simulink model "kb1ram"  (R2020a)
settings: Solver=VariableStepAuto  StartTime=0.0  StopTime=10.0  RelTol=1e-3
libraries: simulink_extras x10
settings Model: Creator=kishan  LastModifiedBy=kishan

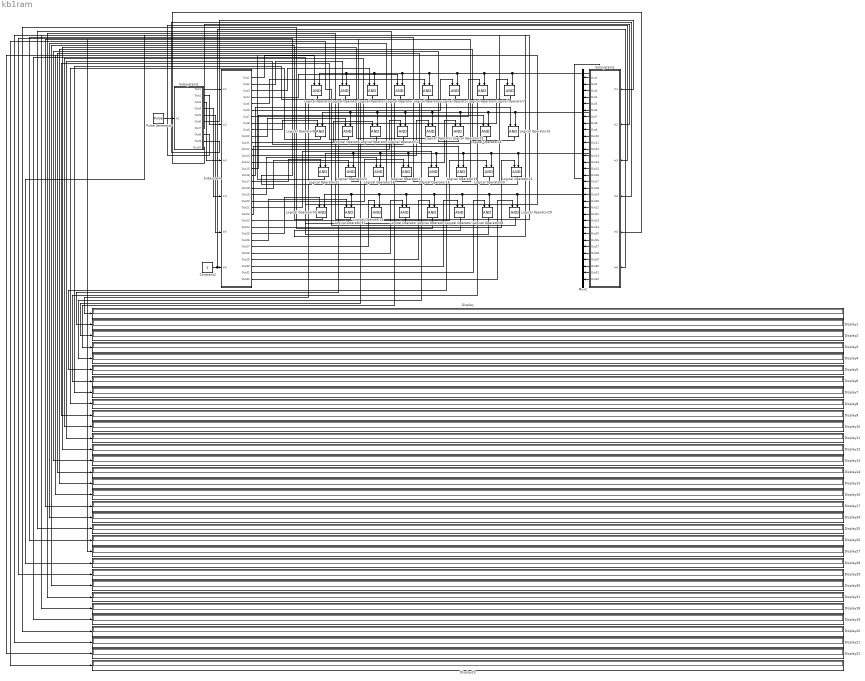
== system kb1ram ==
  Constant2 : Constant
  Display{,1..31} (32 alike) : Display
  Logical Operator{,1..31} (32 alike) : Logic  AllPortsSameDT=off  OutDataTypeStr=boolean
  Mux2 : Mux  Inputs=32
  Pulse Generator : DiscretePulseGenerator  PulseType=Time based  Period=0.005  PulseWidth=5
  Subsystem : Subsystem
  Subsystem1 : Subsystem
  Subsystem2 : Subsystem
  wires:
  Subsystem1/1(Out1) -> Mux2/1
  Subsystem1/2(Out2) -> Mux2/2
  Subsystem1/3(Out3) -> Mux2/3
  Subsystem1/4(Out4) -> Mux2/4
  Subsystem1/5(Out5) -> Mux2/5
  Subsystem1/6(Out6) -> Mux2/6
  Subsystem1/7(Out7) -> Mux2/7
  Subsystem1/8(Out8) -> Mux2/8
  Subsystem1/9(Out9) -> Mux2/9
  Subsystem1/10(Out10) -> Mux2/10
  Subsystem1/11(Out11) -> Mux2/11
  Subsystem1/12(Out12) -> Mux2/12
  Subsystem1/13(Out13) -> Mux2/13
  Subsystem1/14(Out14) -> Mux2/14
  Subsystem1/15(Out15) -> Mux2/15
  Subsystem1/16(Out16) -> Mux2/16
  Subsystem1/17(Out17) -> Mux2/17
  Subsystem1/18(Out18) -> Mux2/18
  Subsystem1/19(Out19) -> Mux2/19
  Subsystem1/20(Out20) -> Mux2/20
  Subsystem1/21(Out21) -> Mux2/21
  Subsystem1/22(Out22) -> Mux2/22
  Subsystem1/23(Out23) -> Mux2/23
  Subsystem1/24(Out24) -> Mux2/24
  Subsystem1/25(Out25) -> Mux2/25
  Subsystem1/26(Out26) -> Mux2/26
  Subsystem1/27(Out27) -> Mux2/27
  Subsystem1/28(Out28) -> Mux2/28
  Subsystem1/29(Out29) -> Mux2/29
  Subsystem1/30(Out30) -> Mux2/30
  Subsystem1/31(Out31) -> Mux2/31
  Subsystem1/32(Out32) -> Mux2/32
  Subsystem2/1(Out1) -> Subsystem/1(In1)
  Subsystem2/2(Out2) -> Subsystem/2(In2)
  Subsystem2/5(Out5) -> Subsystem/5(In5)
  Subsystem2/4(Out4) -> Subsystem/4(In4)
  Subsystem2/3(Out3) -> Subsystem/3(In3)
  Subsystem2/6(Out6) -> Subsystem1/1(In1)
  Subsystem2/7(Out7) -> Subsystem1/2(In2)
  Subsystem2/8(Out8) -> Subsystem1/3(In3)
  Constant2/1 -> Subsystem1/6(In6), Subsystem/6(In6)
  Subsystem2/10(Out10) -> Subsystem1/5(In5)
  Subsystem2/9(Out9) -> Subsystem1/4(In4)
  Subsystem/1(Out1) -> Logical Operator/1
  Subsystem/2(Out2) -> Logical Operator1/1
  Subsystem/3(Out3) -> Logical Operator2/1
  Subsystem/4(Out4) -> Logical Operator3/1
  Mux2/1 -> Logical Operator31/2, Logical Operator30/2, Logical Operator24/2, Logical Operator25/2, Logical Operator26/2, Logical Operator27/2, Logical Operator28/2, Logical Operator29/2, Logical Operator21/2, Logical Operator23/2, Logical Operator22/2, Logical Operator16/2, Logical Operator17/2, Logical Operator18/2, Logical Operator19/2, Logical Operator20/2, Logical Operator9/2, Logical Operator8/2, Logical Operator10/2, Logical Operator11/2, Logical Operator12/2, Logical Operator13/2, Logical Operator14/2, Logical Operator15/2, Logical Operator1/2, Logical Operator/2, Logical Operator2/2, Logical Operator3/2, Logical Operator4/2, Logical Operator5/2, Logical Operator6/2, Logical Operator7/2
  Subsystem/5(Out5) -> Logical Operator4/1
  Subsystem/6(Out6) -> Logical Operator5/1
  Subsystem/7(Out7) -> Logical Operator6/1
  Subsystem/8(Out8) -> Logical Operator7/1
  Subsystem/9(Out9) -> Logical Operator8/1
  Subsystem/10(Out10) -> Logical Operator9/1
  Subsystem/11(Out11) -> Logical Operator10/1
  Subsystem/12(Out12) -> Logical Operator11/1
  Subsystem/13(Out13) -> Logical Operator12/1
  Subsystem/14(Out14) -> Logical Operator13/1
  Subsystem/15(Out15) -> Logical Operator14/1
  Subsystem/16(Out16) -> Logical Operator15/1
  Subsystem/17(Out17) -> Logical Operator22/1
  Subsystem/18(Out18) -> Logical Operator23/1
  Subsystem/19(Out19) -> Logical Operator16/1
  Subsystem/20(Out20) -> Logical Operator17/1
  Subsystem/21(Out21) -> Logical Operator18/1
  Subsystem/22(Out22) -> Logical Operator19/1
  Subsystem/23(Out23) -> Logical Operator20/1
  Subsystem/24(Out24) -> Logical Operator21/1
  Subsystem/25(Out25) -> Logical Operator30/1
  Subsystem/26(Out26) -> Logical Operator31/1
  Subsystem/27(Out27) -> Logical Operator24/1
  Subsystem/28(Out28) -> Logical Operator25/1
  Subsystem/29(Out29) -> Logical Operator26/1
  Subsystem/30(Out30) -> Logical Operator27/1
  Subsystem/31(Out31) -> Logical Operator28/1
  Subsystem/32(Out32) -> Logical Operator29/1
  Logical Operator/1 -> Display/1
  Logical Operator1/1 -> Display1/1
  Logical Operator2/1 -> Display2/1
  Logical Operator3/1 -> Display3/1
  Logical Operator4/1 -> Display4/1
  Logical Operator5/1 -> Display5/1
  Logical Operator6/1 -> Display6/1
  Logical Operator7/1 -> Display7/1
  Logical Operator8/1 -> Display8/1
  Logical Operator9/1 -> Display9/1
  Logical Operator10/1 -> Display10/1
  Logical Operator11/1 -> Display11/1
  Logical Operator12/1 -> Display12/1
  Logical Operator13/1 -> Display13/1
  Logical Operator14/1 -> Display14/1
  Logical Operator15/1 -> Display15/1
  Logical Operator17/1 -> Display25/1
  Logical Operator30/1 -> Display30/1
  Logical Operator22/1 -> Display16/1
  Logical Operator26/1 -> Display20/1
  Logical Operator27/1 -> Display21/1
  Logical Operator18/1 -> Display26/1
  Logical Operator29/1 -> Display23/1
  Logical Operator31/1 -> Display31/1
  Logical Operator25/1 -> Display19/1
  Logical Operator19/1 -> Display27/1
  Logical Operator28/1 -> Display22/1
  Logical Operator21/1 -> Display29/1
  Logical Operator24/1 -> Display18/1
  Logical Operator16/1 -> Display24/1
  Logical Operator20/1 -> Display28/1
  Logical Operator23/1 -> Display17/1
  Pulse Generator/1 -> Subsystem2/1(In1)

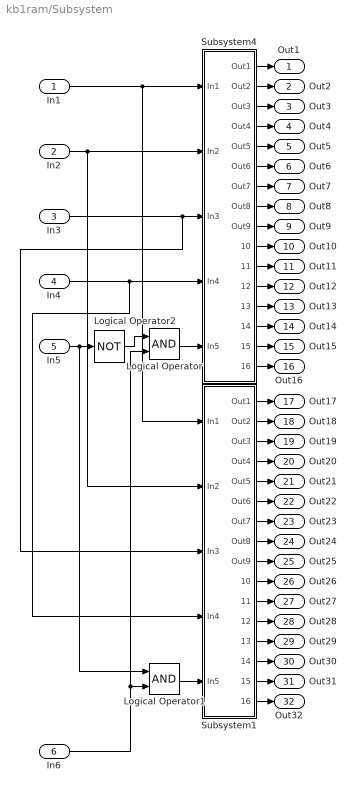
== system kb1ram/Subsystem ==
  In1 : Inport
  In2 : Inport  Port=2
  In3 : Inport  Port=3
  In4 : Inport  Port=4
  In5 : Inport  Port=5
  In6 : Inport  Port=6
  Logical Operator : Logic  AllPortsSameDT=off  OutDataTypeStr=boolean
  Logical Operator1 : Logic  AllPortsSameDT=off  OutDataTypeStr=boolean
  Logical Operator2 : Logic  Operator=NOT  AllPortsSameDT=off  OutDataTypeStr=boolean
  Subsystem1 : Subsystem
  Subsystem4 : Subsystem
  Out1 : Outport
  Out2 : Outport  Port=2
  Out3 : Outport  Port=3
  Out4 : Outport  Port=4
  Out5 : Outport  Port=5
  Out6 : Outport  Port=6
  Out7 : Outport  Port=7
  Out8 : Outport  Port=8
  Out9 : Outport  Port=9
  Out10 : Outport  Port=10
  Out11 : Outport  Port=11
  Out12 : Outport  Port=12
  Out13 : Outport  Port=13
  Out14 : Outport  Port=14
  Out15 : Outport  Port=15
  Out16 : Outport  Port=16
  Out17 : Outport  Port=17
  Out18 : Outport  Port=18
  Out19 : Outport  Port=19
  Out20 : Outport  Port=20
  Out21 : Outport  Port=21
  Out22 : Outport  Port=22
  Out23 : Outport  Port=23
  Out24 : Outport  Port=24
  Out25 : Outport  Port=25
  Out26 : Outport  Port=26
  Out27 : Outport  Port=27
  Out28 : Outport  Port=28
  Out29 : Outport  Port=29
  Out30 : Outport  Port=30
  Out31 : Outport  Port=31
  Out32 : Outport  Port=32
  wires:
  Subsystem1/3(Out3) -> Out19/1
  Subsystem4/2(Out2) -> Out2/1
  Logical Operator2/1 -> Logical Operator/1
  Subsystem4/4(Out4) -> Out4/1
  Subsystem4/11(Out11) -> Out11/1
  Subsystem1/13(Out13) -> Out29/1
  Subsystem4/9(Out9) -> Out9/1
  Subsystem4/13(Out13) -> Out13/1
  Subsystem4/7(Out7) -> Out7/1
  Subsystem1/12(Out12) -> Out28/1
  Subsystem4/6(Out6) -> Out6/1
  Subsystem1/14(Out14) -> Out30/1
  Logical Operator1/1 -> Subsystem1/5(In5)
  Subsystem4/5(Out5) -> Out5/1
  Subsystem1/9(Out9) -> Out25/1
  Subsystem4/10(Out10) -> Out10/1
  Subsystem4/8(Out8) -> Out8/1
  In6/1 -> Logical Operator/2, Logical Operator1/2
  Subsystem1/4(Out4) -> Out20/1
  Subsystem1/15(Out15) -> Out31/1
  In1/1 -> Subsystem4/1(In1), Subsystem1/1(In1)
  Subsystem1/6(Out6) -> Out22/1
  Subsystem1/10(Out10) -> Out26/1
  Subsystem1/11(Out11) -> Out27/1
  Subsystem1/2(Out2) -> Out18/1
  Subsystem1/7(Out7) -> Out23/1
  Subsystem4/1(Out1) -> Out1/1
  Subsystem1/16(Out16) -> Out32/1
  Subsystem1/1(Out1) -> Out17/1
  Subsystem4/12(Out12) -> Out12/1
  In4/1 -> Subsystem1/4(In4), Subsystem4/4(In4)
  Subsystem1/8(Out8) -> Out24/1
  In2/1 -> Subsystem4/2(In2), Subsystem1/2(In2)
  In5/1 -> Logical Operator1/1, Logical Operator2/1
  Subsystem4/3(Out3) -> Out3/1
  Subsystem4/15(Out15) -> Out15/1
  Subsystem4/16(Out16) -> Out16/1
  Subsystem1/5(Out5) -> Out21/1
  Subsystem4/14(Out14) -> Out14/1
  In3/1 -> Subsystem1/3(In3), Subsystem4/3(In3)
  Logical Operator/1 -> Subsystem4/5(In5)

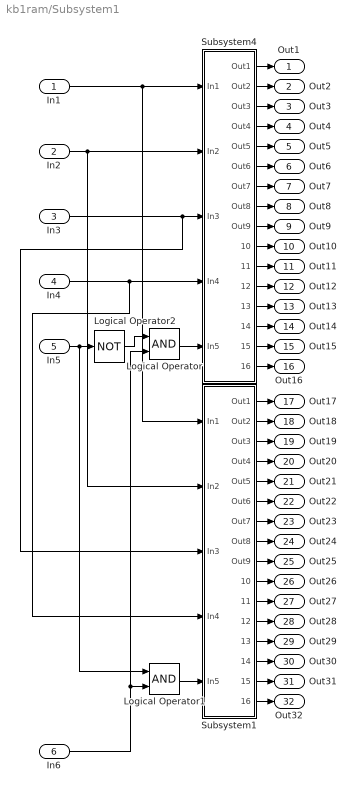
== system kb1ram/Subsystem1 ==
  In1 : Inport
  In2 : Inport  Port=2
  In3 : Inport  Port=3
  In4 : Inport  Port=4
  In5 : Inport  Port=5
  In6 : Inport  Port=6
  Logical Operator : Logic  AllPortsSameDT=off  OutDataTypeStr=boolean
  Logical Operator1 : Logic  AllPortsSameDT=off  OutDataTypeStr=boolean
  Logical Operator2 : Logic  Operator=NOT  AllPortsSameDT=off  OutDataTypeStr=boolean
  Subsystem1 : Subsystem
  Subsystem4 : Subsystem
  Out1 : Outport
  Out2 : Outport  Port=2
  Out3 : Outport  Port=3
  Out4 : Outport  Port=4
  Out5 : Outport  Port=5
  Out6 : Outport  Port=6
  Out7 : Outport  Port=7
  Out8 : Outport  Port=8
  Out9 : Outport  Port=9
  Out10 : Outport  Port=10
  Out11 : Outport  Port=11
  Out12 : Outport  Port=12
  Out13 : Outport  Port=13
  Out14 : Outport  Port=14
  Out15 : Outport  Port=15
  Out16 : Outport  Port=16
  Out17 : Outport  Port=17
  Out18 : Outport  Port=18
  Out19 : Outport  Port=19
  Out20 : Outport  Port=20
  Out21 : Outport  Port=21
  Out22 : Outport  Port=22
  Out23 : Outport  Port=23
  Out24 : Outport  Port=24
  Out25 : Outport  Port=25
  Out26 : Outport  Port=26
  Out27 : Outport  Port=27
  Out28 : Outport  Port=28
  Out29 : Outport  Port=29
  Out30 : Outport  Port=30
  Out31 : Outport  Port=31
  Out32 : Outport  Port=32
  wires:
  Subsystem1/3(Out3) -> Out19/1
  Subsystem4/2(Out2) -> Out2/1
  Logical Operator2/1 -> Logical Operator/1
  Subsystem4/4(Out4) -> Out4/1
  Subsystem4/11(Out11) -> Out11/1
  Subsystem1/13(Out13) -> Out29/1
  Subsystem4/9(Out9) -> Out9/1
  Subsystem4/13(Out13) -> Out13/1
  Subsystem4/7(Out7) -> Out7/1
  Subsystem1/12(Out12) -> Out28/1
  Subsystem4/6(Out6) -> Out6/1
  Subsystem1/14(Out14) -> Out30/1
  Logical Operator1/1 -> Subsystem1/5(In5)
  Subsystem4/5(Out5) -> Out5/1
  Subsystem1/9(Out9) -> Out25/1
  Subsystem4/10(Out10) -> Out10/1
  Subsystem4/8(Out8) -> Out8/1
  In6/1 -> Logical Operator/2, Logical Operator1/2
  Subsystem1/4(Out4) -> Out20/1
  Subsystem1/15(Out15) -> Out31/1
  In1/1 -> Subsystem4/1(In1), Subsystem1/1(In1)
  Subsystem1/6(Out6) -> Out22/1
  Subsystem1/10(Out10) -> Out26/1
  Subsystem1/11(Out11) -> Out27/1
  Subsystem1/2(Out2) -> Out18/1
  Subsystem1/7(Out7) -> Out23/1
  Subsystem4/1(Out1) -> Out1/1
  Subsystem1/16(Out16) -> Out32/1
  Subsystem1/1(Out1) -> Out17/1
  Subsystem4/12(Out12) -> Out12/1
  In4/1 -> Subsystem1/4(In4), Subsystem4/4(In4)
  Subsystem1/8(Out8) -> Out24/1
  In2/1 -> Subsystem4/2(In2), Subsystem1/2(In2)
  In5/1 -> Logical Operator1/1, Logical Operator2/1
  Subsystem4/3(Out3) -> Out3/1
  Subsystem4/15(Out15) -> Out15/1
  Subsystem4/16(Out16) -> Out16/1
  Subsystem1/5(Out5) -> Out21/1
  Subsystem4/14(Out14) -> Out14/1
  In3/1 -> Subsystem1/3(In3), Subsystem4/3(In3)
  Logical Operator/1 -> Subsystem4/5(In5)

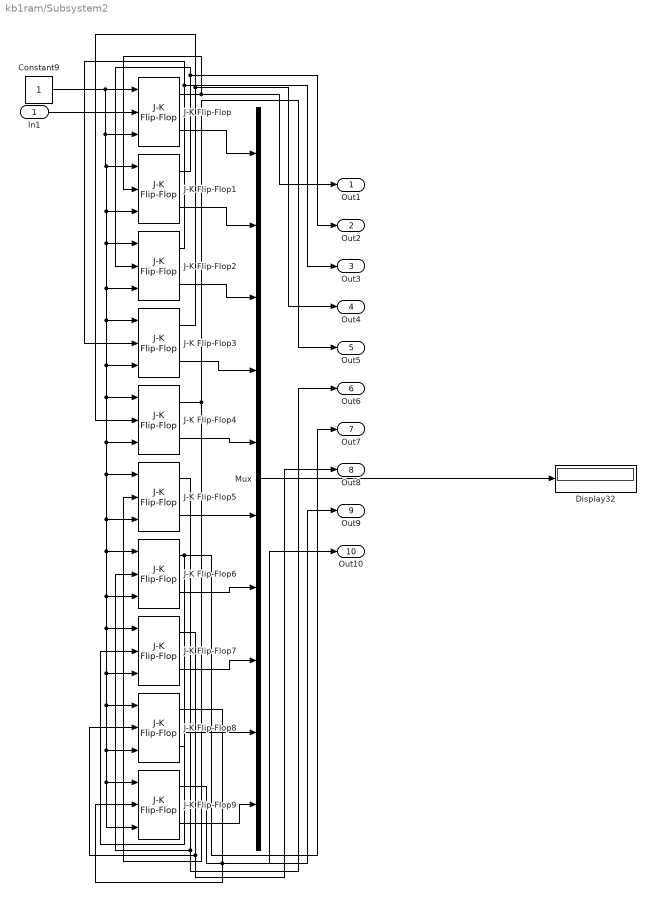
== system kb1ram/Subsystem2 ==
  In1 : Inport
  Constant9 : Constant  OutDataTypeStr=boolean
  Display32 : Display
  J-K Flip-Flop{,1..9} (10 alike) : simulink_extras/Flip Flops/J-K Flip-Flop  initial_condition=0
  Mux : Mux  Inputs=10
  Out1 : Outport
  Out2 : Outport  Port=2
  Out3 : Outport  Port=3
  Out4 : Outport  Port=4
  Out5 : Outport  Port=5
  Out6 : Outport  Port=6
  Out7 : Outport  Port=7
  Out8 : Outport  Port=8
  Out9 : Outport  Port=9
  Out10 : Outport  Port=10
  wires:
  J-K Flip-Flop4/2 -> Mux/5
  J-K Flip-Flop8/1 -> Out9/1, J-K Flip-Flop9/2
  J-K Flip-Flop5/1 -> Out6/1, J-K Flip-Flop6/2
  J-K Flip-Flop3/2 -> Mux/4
  J-K Flip-Flop1/1 -> Out2/1, J-K Flip-Flop2/2
  J-K Flip-Flop/1 -> Out1/1, J-K Flip-Flop1/2
  J-K Flip-Flop3/1 -> Out4/1, J-K Flip-Flop4/2
  J-K Flip-Flop8/2 -> Mux/9
  J-K Flip-Flop6/2 -> Mux/7
  J-K Flip-Flop9/1 -> Out10/1
  J-K Flip-Flop4/1 -> Out5/1, J-K Flip-Flop5/2
  In1/1 -> J-K Flip-Flop/2
  J-K Flip-Flop6/1 -> Out7/1, J-K Flip-Flop7/2
  J-K Flip-Flop2/1 -> J-K Flip-Flop3/2, Out3/1
  J-K Flip-Flop7/1 -> Out8/1, J-K Flip-Flop8/2
  Constant9/1 -> J-K Flip-Flop9/3, J-K Flip-Flop9/1, J-K Flip-Flop8/3, J-K Flip-Flop8/1, J-K Flip-Flop7/3, J-K Flip-Flop7/1, J-K Flip-Flop6/3, J-K Flip-Flop6/1, J-K Flip-Flop5/3, J-K Flip-Flop5/1, J-K Flip-Flop4/3, J-K Flip-Flop4/1, J-K Flip-Flop3/3, J-K Flip-Flop3/1, J-K Flip-Flop2/3, J-K Flip-Flop2/1, J-K Flip-Flop1/3, J-K Flip-Flop1/1, J-K Flip-Flop/3, J-K Flip-Flop/1
  J-K Flip-Flop2/2 -> Mux/3
  J-K Flip-Flop1/2 -> Mux/2
  J-K Flip-Flop5/2 -> Mux/6
  Mux/1 -> Display32/1
  J-K Flip-Flop/2 -> Mux/1
  J-K Flip-Flop7/2 -> Mux/8
  J-K Flip-Flop9/2 -> Mux/10

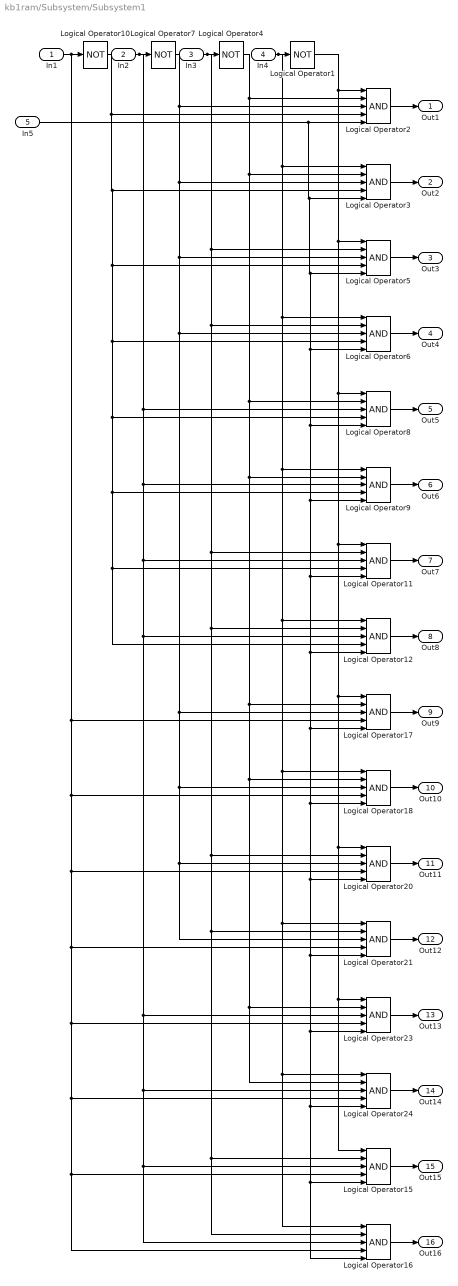
== system kb1ram/Subsystem/Subsystem1 ==
  In1 : Inport
  In2 : Inport  Port=2
  In3 : Inport  Port=3
  In4 : Inport  Port=4
  In5 : Inport  Port=5
  Logical Operator{1,4,7,10} (4 alike) : Logic  Operator=NOT  AllPortsSameDT=off  OutDataTypeStr=boolean
  Logical Operator{2..3,5..6,8..9,11..12,15..18,20..21,23..24} (16 alike) : Logic  Inputs=5  AllPortsSameDT=off  OutDataTypeStr=boolean
  Out1 : Outport
  Out2 : Outport  Port=2
  Out3 : Outport  Port=3
  Out4 : Outport  Port=4
  Out5 : Outport  Port=5
  Out6 : Outport  Port=6
  Out7 : Outport  Port=7
  Out8 : Outport  Port=8
  Out9 : Outport  Port=9
  Out10 : Outport  Port=10
  Out11 : Outport  Port=11
  Out12 : Outport  Port=12
  Out13 : Outport  Port=13
  Out14 : Outport  Port=14
  Out15 : Outport  Port=15
  Out16 : Outport  Port=16
  wires:
  Logical Operator11/1 -> Out7/1
  Logical Operator12/1 -> Out8/1
  Logical Operator18/1 -> Out10/1
  In2/1 -> Logical Operator16/3, Logical Operator15/3, Logical Operator24/3, Logical Operator23/3, Logical Operator12/3, Logical Operator11/3, Logical Operator9/3, Logical Operator8/3, Logical Operator7/1
  In3/1 -> Logical Operator11/2, Logical Operator15/2, Logical Operator16/2, Logical Operator21/2, Logical Operator20/2, Logical Operator12/2, Logical Operator6/2, Logical Operator5/2, Logical Operator4/1
  Logical Operator24/1 -> Out14/1
  In4/1 -> Logical Operator16/1, Logical Operator24/1, Logical Operator21/1, Logical Operator18/1, Logical Operator12/1, Logical Operator9/1, Logical Operator6/1, Logical Operator3/1, Logical Operator1/1
  Logical Operator10/1 -> Logical Operator12/4, Logical Operator11/4, Logical Operator9/4, Logical Operator8/4, Logical Operator6/4, Logical Operator5/4, Logical Operator3/4, Logical Operator2/4
  Logical Operator9/1 -> Out6/1
  In5/1 -> Logical Operator16/5, Logical Operator15/5, Logical Operator24/5, Logical Operator23/5, Logical Operator21/5, Logical Operator20/5, Logical Operator18/5, Logical Operator17/5, Logical Operator12/5, Logical Operator11/5, Logical Operator9/5, Logical Operator8/5, Logical Operator6/5, Logical Operator5/5, Logical Operator3/5, Logical Operator2/5
  Logical Operator5/1 -> Out3/1
  Logical Operator1/1 -> Logical Operator15/1, Logical Operator23/1, Logical Operator20/1, Logical Operator17/1, Logical Operator11/1, Logical Operator8/1, Logical Operator5/1, Logical Operator2/1
  Logical Operator2/1 -> Out1/1
  Logical Operator21/1 -> Out12/1
  Logical Operator8/1 -> Out5/1
  Logical Operator7/1 -> Logical Operator21/3, Logical Operator20/3, Logical Operator18/3, Logical Operator17/3, Logical Operator6/3, Logical Operator5/3, Logical Operator3/3, Logical Operator2/3
  Logical Operator16/1 -> Out16/1
  Logical Operator15/1 -> Out15/1
  In1/1 -> Logical Operator17/4, Logical Operator18/4, Logical Operator20/4, Logical Operator21/4, Logical Operator23/4, Logical Operator24/4, Logical Operator15/4, Logical Operator16/4, Logical Operator10/1
  Logical Operator3/1 -> Out2/1
  Logical Operator20/1 -> Out11/1
  Logical Operator6/1 -> Out4/1
  Logical Operator23/1 -> Out13/1
  Logical Operator4/1 -> Logical Operator24/2, Logical Operator23/2, Logical Operator18/2, Logical Operator17/2, Logical Operator9/2, Logical Operator8/2, Logical Operator3/2, Logical Operator2/2
  Logical Operator17/1 -> Out9/1

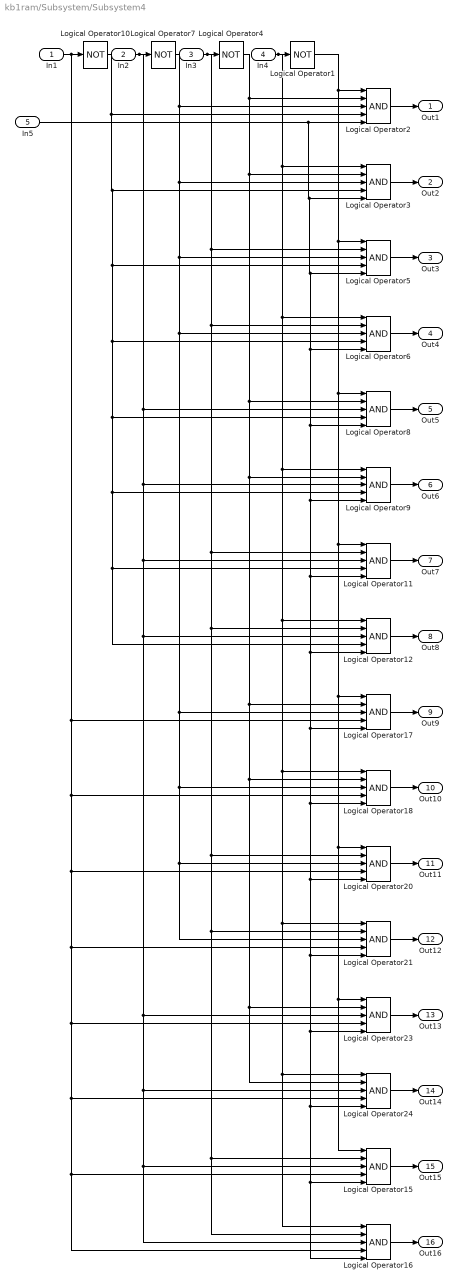
== system kb1ram/Subsystem/Subsystem4 ==
  In1 : Inport
  In2 : Inport  Port=2
  In3 : Inport  Port=3
  In4 : Inport  Port=4
  In5 : Inport  Port=5
  Logical Operator{1,4,7,10} (4 alike) : Logic  Operator=NOT  AllPortsSameDT=off  OutDataTypeStr=boolean
  Logical Operator{2..3,5..6,8..9,11..12,15..18,20..21,23..24} (16 alike) : Logic  Inputs=5  AllPortsSameDT=off  OutDataTypeStr=boolean
  Out1 : Outport
  Out2 : Outport  Port=2
  Out3 : Outport  Port=3
  Out4 : Outport  Port=4
  Out5 : Outport  Port=5
  Out6 : Outport  Port=6
  Out7 : Outport  Port=7
  Out8 : Outport  Port=8
  Out9 : Outport  Port=9
  Out10 : Outport  Port=10
  Out11 : Outport  Port=11
  Out12 : Outport  Port=12
  Out13 : Outport  Port=13
  Out14 : Outport  Port=14
  Out15 : Outport  Port=15
  Out16 : Outport  Port=16
  wires:
  Logical Operator11/1 -> Out7/1
  Logical Operator12/1 -> Out8/1
  Logical Operator18/1 -> Out10/1
  In2/1 -> Logical Operator16/3, Logical Operator15/3, Logical Operator24/3, Logical Operator23/3, Logical Operator12/3, Logical Operator11/3, Logical Operator9/3, Logical Operator8/3, Logical Operator7/1
  In3/1 -> Logical Operator11/2, Logical Operator15/2, Logical Operator16/2, Logical Operator21/2, Logical Operator20/2, Logical Operator12/2, Logical Operator6/2, Logical Operator5/2, Logical Operator4/1
  Logical Operator24/1 -> Out14/1
  In4/1 -> Logical Operator16/1, Logical Operator24/1, Logical Operator21/1, Logical Operator18/1, Logical Operator12/1, Logical Operator9/1, Logical Operator6/1, Logical Operator3/1, Logical Operator1/1
  Logical Operator10/1 -> Logical Operator12/4, Logical Operator11/4, Logical Operator9/4, Logical Operator8/4, Logical Operator6/4, Logical Operator5/4, Logical Operator3/4, Logical Operator2/4
  Logical Operator9/1 -> Out6/1
  In5/1 -> Logical Operator16/5, Logical Operator15/5, Logical Operator24/5, Logical Operator23/5, Logical Operator21/5, Logical Operator20/5, Logical Operator18/5, Logical Operator17/5, Logical Operator12/5, Logical Operator11/5, Logical Operator9/5, Logical Operator8/5, Logical Operator6/5, Logical Operator5/5, Logical Operator3/5, Logical Operator2/5
  Logical Operator5/1 -> Out3/1
  Logical Operator1/1 -> Logical Operator15/1, Logical Operator23/1, Logical Operator20/1, Logical Operator17/1, Logical Operator11/1, Logical Operator8/1, Logical Operator5/1, Logical Operator2/1
  Logical Operator2/1 -> Out1/1
  Logical Operator21/1 -> Out12/1
  Logical Operator8/1 -> Out5/1
  Logical Operator7/1 -> Logical Operator21/3, Logical Operator20/3, Logical Operator18/3, Logical Operator17/3, Logical Operator6/3, Logical Operator5/3, Logical Operator3/3, Logical Operator2/3
  Logical Operator16/1 -> Out16/1
  Logical Operator15/1 -> Out15/1
  In1/1 -> Logical Operator17/4, Logical Operator18/4, Logical Operator20/4, Logical Operator21/4, Logical Operator23/4, Logical Operator24/4, Logical Operator15/4, Logical Operator16/4, Logical Operator10/1
  Logical Operator3/1 -> Out2/1
  Logical Operator20/1 -> Out11/1
  Logical Operator6/1 -> Out4/1
  Logical Operator23/1 -> Out13/1
  Logical Operator4/1 -> Logical Operator24/2, Logical Operator23/2, Logical Operator18/2, Logical Operator17/2, Logical Operator9/2, Logical Operator8/2, Logical Operator3/2, Logical Operator2/2
  Logical Operator17/1 -> Out9/1

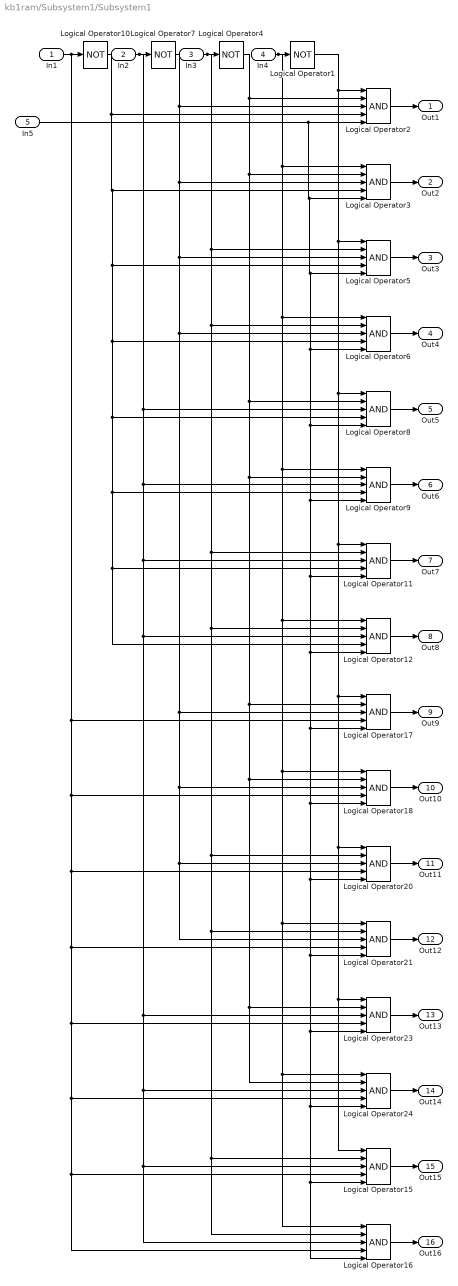
== system kb1ram/Subsystem1/Subsystem1 ==
  In1 : Inport
  In2 : Inport  Port=2
  In3 : Inport  Port=3
  In4 : Inport  Port=4
  In5 : Inport  Port=5
  Logical Operator{1,4,7,10} (4 alike) : Logic  Operator=NOT  AllPortsSameDT=off  OutDataTypeStr=boolean
  Logical Operator{2..3,5..6,8..9,11..12,15..18,20..21,23..24} (16 alike) : Logic  Inputs=5  AllPortsSameDT=off  OutDataTypeStr=boolean
  Out1 : Outport
  Out2 : Outport  Port=2
  Out3 : Outport  Port=3
  Out4 : Outport  Port=4
  Out5 : Outport  Port=5
  Out6 : Outport  Port=6
  Out7 : Outport  Port=7
  Out8 : Outport  Port=8
  Out9 : Outport  Port=9
  Out10 : Outport  Port=10
  Out11 : Outport  Port=11
  Out12 : Outport  Port=12
  Out13 : Outport  Port=13
  Out14 : Outport  Port=14
  Out15 : Outport  Port=15
  Out16 : Outport  Port=16
  wires:
  Logical Operator11/1 -> Out7/1
  Logical Operator12/1 -> Out8/1
  Logical Operator18/1 -> Out10/1
  In2/1 -> Logical Operator16/3, Logical Operator15/3, Logical Operator24/3, Logical Operator23/3, Logical Operator12/3, Logical Operator11/3, Logical Operator9/3, Logical Operator8/3, Logical Operator7/1
  In3/1 -> Logical Operator11/2, Logical Operator15/2, Logical Operator16/2, Logical Operator21/2, Logical Operator20/2, Logical Operator12/2, Logical Operator6/2, Logical Operator5/2, Logical Operator4/1
  Logical Operator24/1 -> Out14/1
  In4/1 -> Logical Operator16/1, Logical Operator24/1, Logical Operator21/1, Logical Operator18/1, Logical Operator12/1, Logical Operator9/1, Logical Operator6/1, Logical Operator3/1, Logical Operator1/1
  Logical Operator10/1 -> Logical Operator12/4, Logical Operator11/4, Logical Operator9/4, Logical Operator8/4, Logical Operator6/4, Logical Operator5/4, Logical Operator3/4, Logical Operator2/4
  Logical Operator9/1 -> Out6/1
  In5/1 -> Logical Operator16/5, Logical Operator15/5, Logical Operator24/5, Logical Operator23/5, Logical Operator21/5, Logical Operator20/5, Logical Operator18/5, Logical Operator17/5, Logical Operator12/5, Logical Operator11/5, Logical Operator9/5, Logical Operator8/5, Logical Operator6/5, Logical Operator5/5, Logical Operator3/5, Logical Operator2/5
  Logical Operator5/1 -> Out3/1
  Logical Operator1/1 -> Logical Operator15/1, Logical Operator23/1, Logical Operator20/1, Logical Operator17/1, Logical Operator11/1, Logical Operator8/1, Logical Operator5/1, Logical Operator2/1
  Logical Operator2/1 -> Out1/1
  Logical Operator21/1 -> Out12/1
  Logical Operator8/1 -> Out5/1
  Logical Operator7/1 -> Logical Operator21/3, Logical Operator20/3, Logical Operator18/3, Logical Operator17/3, Logical Operator6/3, Logical Operator5/3, Logical Operator3/3, Logical Operator2/3
  Logical Operator16/1 -> Out16/1
  Logical Operator15/1 -> Out15/1
  In1/1 -> Logical Operator17/4, Logical Operator18/4, Logical Operator20/4, Logical Operator21/4, Logical Operator23/4, Logical Operator24/4, Logical Operator15/4, Logical Operator16/4, Logical Operator10/1
  Logical Operator3/1 -> Out2/1
  Logical Operator20/1 -> Out11/1
  Logical Operator6/1 -> Out4/1
  Logical Operator23/1 -> Out13/1
  Logical Operator4/1 -> Logical Operator24/2, Logical Operator23/2, Logical Operator18/2, Logical Operator17/2, Logical Operator9/2, Logical Operator8/2, Logical Operator3/2, Logical Operator2/2
  Logical Operator17/1 -> Out9/1

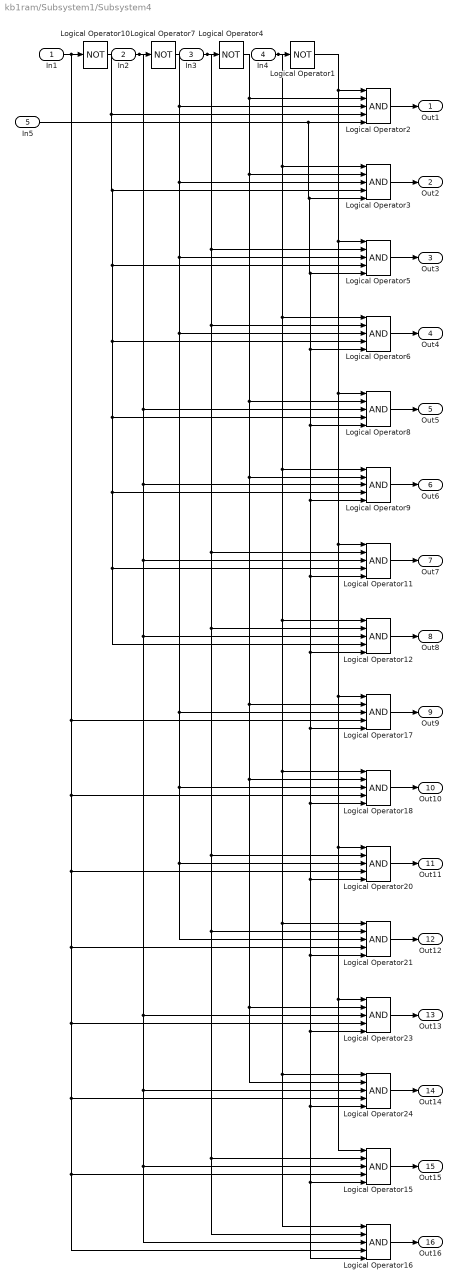
== system kb1ram/Subsystem1/Subsystem4 ==
  In1 : Inport
  In2 : Inport  Port=2
  In3 : Inport  Port=3
  In4 : Inport  Port=4
  In5 : Inport  Port=5
  Logical Operator{1,4,7,10} (4 alike) : Logic  Operator=NOT  AllPortsSameDT=off  OutDataTypeStr=boolean
  Logical Operator{2..3,5..6,8..9,11..12,15..18,20..21,23..24} (16 alike) : Logic  Inputs=5  AllPortsSameDT=off  OutDataTypeStr=boolean
  Out1 : Outport
  Out2 : Outport  Port=2
  Out3 : Outport  Port=3
  Out4 : Outport  Port=4
  Out5 : Outport  Port=5
  Out6 : Outport  Port=6
  Out7 : Outport  Port=7
  Out8 : Outport  Port=8
  Out9 : Outport  Port=9
  Out10 : Outport  Port=10
  Out11 : Outport  Port=11
  Out12 : Outport  Port=12
  Out13 : Outport  Port=13
  Out14 : Outport  Port=14
  Out15 : Outport  Port=15
  Out16 : Outport  Port=16
  wires:
  Logical Operator11/1 -> Out7/1
  Logical Operator12/1 -> Out8/1
  Logical Operator18/1 -> Out10/1
  In2/1 -> Logical Operator16/3, Logical Operator15/3, Logical Operator24/3, Logical Operator23/3, Logical Operator12/3, Logical Operator11/3, Logical Operator9/3, Logical Operator8/3, Logical Operator7/1
  In3/1 -> Logical Operator11/2, Logical Operator15/2, Logical Operator16/2, Logical Operator21/2, Logical Operator20/2, Logical Operator12/2, Logical Operator6/2, Logical Operator5/2, Logical Operator4/1
  Logical Operator24/1 -> Out14/1
  In4/1 -> Logical Operator16/1, Logical Operator24/1, Logical Operator21/1, Logical Operator18/1, Logical Operator12/1, Logical Operator9/1, Logical Operator6/1, Logical Operator3/1, Logical Operator1/1
  Logical Operator10/1 -> Logical Operator12/4, Logical Operator11/4, Logical Operator9/4, Logical Operator8/4, Logical Operator6/4, Logical Operator5/4, Logical Operator3/4, Logical Operator2/4
  Logical Operator9/1 -> Out6/1
  In5/1 -> Logical Operator16/5, Logical Operator15/5, Logical Operator24/5, Logical Operator23/5, Logical Operator21/5, Logical Operator20/5, Logical Operator18/5, Logical Operator17/5, Logical Operator12/5, Logical Operator11/5, Logical Operator9/5, Logical Operator8/5, Logical Operator6/5, Logical Operator5/5, Logical Operator3/5, Logical Operator2/5
  Logical Operator5/1 -> Out3/1
  Logical Operator1/1 -> Logical Operator15/1, Logical Operator23/1, Logical Operator20/1, Logical Operator17/1, Logical Operator11/1, Logical Operator8/1, Logical Operator5/1, Logical Operator2/1
  Logical Operator2/1 -> Out1/1
  Logical Operator21/1 -> Out12/1
  Logical Operator8/1 -> Out5/1
  Logical Operator7/1 -> Logical Operator21/3, Logical Operator20/3, Logical Operator18/3, Logical Operator17/3, Logical Operator6/3, Logical Operator5/3, Logical Operator3/3, Logical Operator2/3
  Logical Operator16/1 -> Out16/1
  Logical Operator15/1 -> Out15/1
  In1/1 -> Logical Operator17/4, Logical Operator18/4, Logical Operator20/4, Logical Operator21/4, Logical Operator23/4, Logical Operator24/4, Logical Operator15/4, Logical Operator16/4, Logical Operator10/1
  Logical Operator3/1 -> Out2/1
  Logical Operator20/1 -> Out11/1
  Logical Operator6/1 -> Out4/1
  Logical Operator23/1 -> Out13/1
  Logical Operator4/1 -> Logical Operator24/2, Logical Operator23/2, Logical Operator18/2, Logical Operator17/2, Logical Operator9/2, Logical Operator8/2, Logical Operator3/2, Logical Operator2/2
  Logical Operator17/1 -> Out9/1
